simulink model "sim11ex6"  (Simulink 2.09)
settings: Solver=ode45  StartTime=0.0  StopTime=2  MaxStep=.01  RelTol=1e-3  AbsTol=1e-3
settings Model: SaveTime=off  SaveOutput=off  ConsistencyChecking=off  RTWTemplateMakefile=grt_vc.tmf

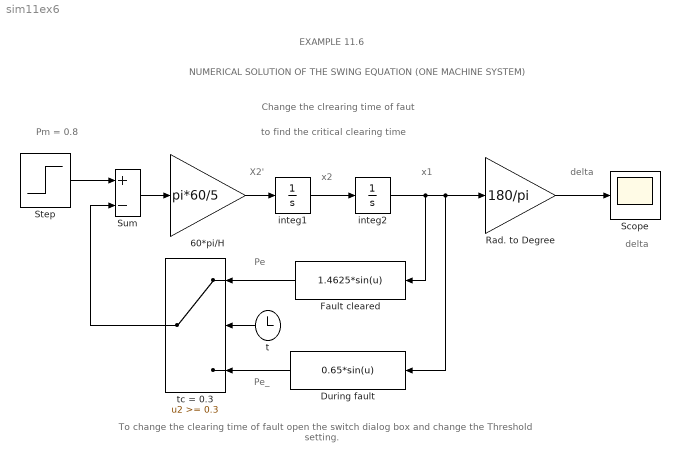
== system sim11ex6 ==
  note: delta
  note: EXAMPLE 11.6
  note: NUMERICAL SOLUTION OF THE SWING EQUATION (ONE MACHINE SYSTEM)
  note: Change the clrearing time of faut
  note: to find the critical clearing time
  note: X2'
  note: x2
  note: Pe
  note: Pe_
  note: x1
  note: delta
  note: To change the clearing time of fault open the switch
      | dialog box and change the Threshold setting.
  note: Pm = 0.8
  " Fault cleared " : Fcn  Orientation=left  Expr=1.4625*sin(u)
  60*pi/H : Gain  Gain=pi*60/5
  During fault : Fcn  Orientation=left  Expr=0.65*sin(u)
  "Rad. to Degree " : Gain  Gain=180/pi
  Scope : Scope
      settings: TickLabels=on  TimeRange=auto  YMin=-5  YMax=5  SaveToWorkspace=off  SaveName=ScopeData
  Step : Step  Time=.01  Before=0.8  After=0.8
  Sum : Sum  Inputs=+-
  integ1 : Integrator  ExternalReset=none  InitialConditionSource=internal  InitialCondition=0  LimitOutput=off  UpperSaturationLimit=inf  LowerSaturationLimit=-inf  ShowSaturationPort=off  ShowStatePort=off  AbsoluteTolerance=auto
  integ2 : Integrator  ExternalReset=none  InitialConditionSource=internal  InitialCondition=0.46055  LimitOutput=off  UpperSaturationLimit=inf  LowerSaturationLimit=-inf  ShowSaturationPort=off  ShowStatePort=off  AbsoluteTolerance=auto
  t : Clock
  tc = 0.3 : Switch  Orientation=left  Threshold=0.3
  wires:
  integ1/1 -> integ2/1
  Step/1 -> Sum/1
  "Rad. to Degree "/1 -> Scope/1
  Sum/1 -> 60*pi/H/1
  60*pi/H/1 -> integ1/1
  " Fault cleared "/1 -> tc = 0.3/1
  During fault/1 -> tc = 0.3/3
  tc = 0.3/1 -> Sum/2
  t/1 -> tc = 0.3/2
  integ2/1 -> " Fault cleared "/1, "Rad. to Degree "/1, During fault/1
